simulink model "Final_EWASP_VC"  (R2022a)
settings: Solver=ode1  StartTime=0.0  StopTime=24*3600  FixedStep=10  RelTol=1e-3
values from neighbouring files (symbols this model uses):
  Aux_Threshold = 52    [Setup_Code_EWASP_VC.m]
  buildingAge = 2005    [Setup_Code_EWASP_VC.m]
  ceilingHeight = 2.4    [Setup_Code_EWASP_VC.m]
  conductiveHconnectMatrix = [ ... (first row only)    [Setup_Code_EWASP_VC.m]
  cRoofGreen = 100000    [Setup_Code_EWASP_VC.m]
  Defrost_After_Time = 30    [Setup_Code_EWASP_VC.m]
  DHWDemandProfile = occFreegainHotwaterElecTestPassiveOcc3(:,3)    [Setup_Code_EWASP_VC.m]
  Elec_Max = Elec_Max*(30/24.2)    [Setup_Code_EWASP_VC.m]
  Elec_Mid = Elec_Mid*(30/24.2)    [Setup_Code_EWASP_VC.m]
  Elec_Min = Elec_Min*(30/24.2)    [Setup_Code_EWASP_VC.m]
  ElecDemandProfile = occFreegainHotwaterElecTestPassiveOcc3(:,4)    [Setup_Code_EWASP_VC.m]
  ElecFixed = [Elec_Max(6,2) Elec_Max(6,4) Elec_Max(6,6) Elec_Max(6,7) ... (first row only)    [Setup_Code_EWASP_VC.m]
  floorOrCeilingArea = floorOrCeilingArea*1.15    [Setup_Code_EWASP_VC.m]
  forceCold = 0    [Setup_Code_EWASP_VC.m]
  freegain = occFreegainHotwaterElecTestPassiveOcc3(:,2)-max(occupancy)*25    [Setup_Code_EWASP_VC.m]
  furnitureModelOn = 1    [Setup_Code_EWASP_VC.m]
  Heat_Max = Heat_Max*(30/24.2)    [Setup_Code_EWASP_VC.m]
  Heat_Mid = Heat_Mid*(30/24.2)    [Setup_Code_EWASP_VC.m]
  Heat_Min = Heat_Min*(30/24.2)    [Setup_Code_EWASP_VC.m]
  HeatFixed = [Heat_Max(6,2) Heat_Max(6,4) Heat_Max(6,6) Heat_Max(6,7) ... (first row only)    [Setup_Code_EWASP_VC.m]
  HeatingOnProfile = repmat(HeatingOnProfile,365,1)    [Setup_Code_EWASP_VC.m]
  HEX_ReturnLowerLimit = 52.5    [Setup_Code_EWASP_VC.m]
  HEX_ReturnUpperLimit = 55    [Setup_Code_EWASP_VC.m]
  LeakMultiplier = 1+(2*(rand()-0.5)/10)    [Setup_Code_EWASP_VC.m]
  loopCap = 15    [Setup_Code_EWASP_VC.m]
  maxOcc = max(occupancyProfile)    [Setup_Code_EWASP_VC.m]
  NESW_wallArea = max(NESW_Lengths*ceilingHeight-NESW_Windows,0)    [Setup_Code_EWASP_VC.m]
  NESW_Windows = [ ... (first row only)    [Setup_Code_EWASP_VC.m]
  numRooms = roomCount    [Setup_Code_EWASP_VC.m]
  offsetDays = 0    [Setup_Code_EWASP_VC.m]
  pumpChoice = pumpChoices(MinIndex,1)    [Setup_Code_EWASP_VC.m]
  pumpRamp = 180    [Setup_Code_EWASP_VC.m]
  ReturnLowerLimit = 37.5    [Setup_Code_EWASP_VC.m]
  ReturnUpperLimit = 40    [Setup_Code_EWASP_VC.m]
  RoofIrradiance = Flat_NS_EW_RoofIrradiance(:,1)    [Setup_Code_EWASP_VC.m]
  roofStartTemp = ones(11,1)*20    [Setup_Code_EWASP_VC.m]
  rooftype = 0    [Setup_Code_EWASP_VC.m]
  RoomDataMatrix = [zeros(1,12);ones(1,12)*wallDensity;zeros(1,12);ones(1,12)*wallU;ones(1,12)*windowU;ones(1,12)*floorU;ones(1,12)*ceilingU;zeros(1,12);windowArea, 0;floorOrCeilingArea;zeros(1,12);floorOrCeilingArea*ceilingHeight]    [Setup_Code_EWASP_VC.m]
  roomVol = roomVol*1.15    [Setup_Code_EWASP_VC.m]
  slabStartTemp = (GroundTempTimeSeries(offsetDays*1440+1,1)+thermostatSetting)/2    [Setup_Code_EWASP_VC.m]
  SlackRequest = zeros(1440,1)    [Setup_Code_EWASP_VC.m]
  SolarThermalExists = 0    [Setup_Code_EWASP_VC.m]
  SourceFixed = HeatFixed-ElecFixed    [Setup_Code_EWASP_VC.m]
  StateSeries = StateSeriesGenerator(22,7,1)    [Setup_Code_EWASP_VC.m]
  Tank_Lower_Temp = 49.5    [Setup_Code_EWASP_VC.m]
  Tank_Upper_Temp = 52    [Setup_Code_EWASP_VC.m]
  Tank_Volume_m3 = 0.15    [Setup_Code_EWASP_VC.m]
  TankHeatHour = randi([1 5])-1    [Setup_Code_EWASP_VC.m]
  thermostatSetting = 20.0    (= 20)    [Setup_Code_EWASP_VC.m]
  upDown = [0;0;0;0;1;1;1;1;1;1;1]    [Setup_Code_EWASP_VC.m]
  variableASHP = 1    [Setup_Code_EWASP_VC.m]
  wallStartTempExt = thermostatSetting*(0.266+0.00215*outdoorStartTemp+0.018*wallU+0.00113*outdoorStartTemp*wallU+0.0068*wallU^2)    [Setup_Code_EWASP_VC.m]
undefined symbols (not defined in the file or in its folder): a, ceilingU, condUDMatrix, convUDMatrix, deltaPEXPANDED_E, deltaPEXPANDED_E2, deltaPEXPANDED_N, deltaPEXPANDED_N2, deltaPEXPANDED_S, deltaPEXPANDED_S2, deltaPEXPANDED_W, deltaPEXPANDED_W2, DesiredDHWTemp, DesiredFlowTempVsInOutDeltaTemp, DiffuseHorizontal, DiscIntNeverNeededParam, DNI, dwnAndConcrete, DWORK_A_HX, DWORK_CHK_FLU, DWORK_CP_NODE, DWORK_DH, DWORK_FLUID, DWORK_HCON, DWORK_LOSS, DWORK_MDOTDOWN, DWORK_MDOTIN, DWORK_MDOTUP, DWORK_MIX, DWORK_PRESS, DWORK_QDOTIN, DWORK_RHO_NODE, DWORK_TIN, DWORK_TS_OLD, DWORK_V_NODE, GroundTempTimeSeries, HCM, HCM2, HCM_closed, HCM_closed2, intermediateU, IsTop, massFlowMatrix, neighbourMatrix, numericalRoomUse, RadiatorMatrix, room2roomflowmatrix_E, room2roomflowmatrix_E2, room2roomflowmatrix_N, room2roomflowmatrix_N2, room2roomflowmatrix_S, room2roomflowmatrix_S2, room2roomflowmatrix_W, room2roomflowmatrix_W2, StateAirInEXPANDED_E, StateAirInEXPANDED_E2, StateAirInEXPANDED_N, StateAirInEXPANDED_N2, StateAirInEXPANDED_S, StateAirInEXPANDED_S2 ... (+23)
libraries: simulink x6, dspsigops x4, dspmtrx3 x4, carnot x3, spsEdgeDetectorLib x2, dspstat3 x2, powerlib_meascontrol x1, simulink_extras x1
(part 23 of 27)

== system Final_EWASP_VC/ASHP_Subsystem_Variable/DHW for ASHP Case/HeatPump_Simplified2/HeatPump_basic/model hot side ==
  note: Qdot_h = K1*Tcold_in + K2*Thot_out + K3
      |
      | Qdot_c = -K7*Tcold_in - K8*Thot_out - K9
      |
      | cap_h*dTh/dt = Qdot_h + mdot_h*cp_h*(Th_in-Th) + UA*(Tamb-Th)
      |
      | cap_c*dTc/dt = Qdot_c + mdot_c*cp_c*(Tc_in-Tc) + UA*(Tamb-Tc)
      |
      | cap_h = mass_hot_side * heat_capactiy_hot_side
      |
      | cap_c = mass_cold_side * heat_capactiy_cold_side
  Tcold : Inport
  Thot : Inport  Port=2
  mdot_hot : Inport  Port=3
  Tamb : Inport  Port=4
  command : Inport  Port=5
  Defrost Delta In : Inport  Port=6
  1/(m*cp) : Gain  Gain=1/caph
  Add1 : Sum
  Add2 : Sum  Inputs=+-
  Add4 : Sum  Inputs=+-
  Bias : Bias  Bias=1  SaturateOnIntegerOverflow=off
  Constant : Constant  Value=4180
  Constant1 : Constant  Value=50
  Discrete-Time Integrator : DiscreteIntegrator  InitialConditionSource=external  SampleTime=-1  ICPrevOutput=DiscIntNeverNeededParam  ICPrevScaledInput=DiscIntNeverNeededParam
  Display{,1..5} (6 alike) : Display
  Product{2..5} (4 alike) : DotProduct  OutDataTypeStr=Inherit: Inherit via internal rule
  Scope : Scope
  Scope1 : Scope
  Sum1 : Sum  Inputs=+++  InputSameDT=on  SaturateOnIntegerOverflow=on  OutDataTypeStr=Inherit: Same as first input
  Sum2 : Sum  Inputs=+++  InputSameDT=on  SaturateOnIntegerOverflow=on  OutDataTypeStr=Inherit: Same as first input
  Thot_dependancy : Gain  Gain=K(2)  SaturateOnIntegerOverflow=on  OutDataTypeStr=Inherit: Same as input  ParamDataTypeStr=Inherit: Same as input
  Tsource dependancy : Gain  Gain=K(1)  SaturateOnIntegerOverflow=on  OutDataTypeStr=Inherit: Same as input  ParamDataTypeStr=Inherit: Same as input
  const Power1 : Gain  Gain=-1  SaturateOnIntegerOverflow=on  OutDataTypeStr=Inherit: Same as input  ParamDataTypeStr=Inherit: Same as input
  constant power : Constant  Value=K(3)
  losses : Gain  Gain=UA
  mdot*cp : Outport  VectorParamsAs1DForOutWhenUnconnected=off
  Thot_out : Outport  Port=2  VectorParamsAs1DForOutWhenUnconnected=off
  Real P_therm : Outport  Port=3  VectorParamsAs1DForOutWhenUnconnected=off
  Main Delta : Outport  Port=4  VectorParamsAs1DForOutWhenUnconnected=off
  wires:
  Thot/1 -> Display1/1, Add4/1
  Product2/1 -> mdot*cp/1, Product5/1
  Constant/1 -> Product2/2
  mdot_hot/1 -> Display/1, Product2/1
  Add2/1 -> losses/1
  Tcold/1 -> Display3/1, Tsource dependancy/1
  Tsource dependancy/1 -> Sum1/1
  Thot_dependancy/1 -> Sum1/2
  constant power/1 -> Sum1/3
  Sum1/1 -> Display5/1, Product4/2  "Qdot_hot"
  Tamb/1 -> Display4/1, Add2/1
  command/1 -> Display2/1, Product4/1, const Power1/1
  losses/1 -> Product3/2
  Bias/1 -> Product3/1
  const Power1/1 -> Bias/1
  Add4/1 -> Product5/2
  Sum2/1 -> 1/(m*cp)/1
  Product3/1 -> Sum2/3
  Product4/1 -> Real P_therm/1, Sum2/2
  Product5/1 -> Sum2/1
  Discrete-Time Integrator/1 -> Thot_out/1, Add4/2, Thot_dependancy/1, Add2/2, Scope/1
  1/(m*cp)/1 -> Add1/1, Main Delta/1, Scope1/1
  Add1/1 -> Discrete-Time Integrator/1
  Defrost Delta In/1 -> Add1/2
  Constant1/1 -> Discrete-Time Integrator/2

== system Final_EWASP_VC/ASHP_Subsystem_Variable/DHW for ASHP Case/Storage_Type_2_CONF/HX_EN12977_1/sfun_storage_heatexchanger ==
  Tnodes : Inport
  Temperature : Inport  Port=2
  MassFlow : Inport  Port=3
  Ground : Ground
  Ground1 : Ground
  Ground2 : Ground
  Mux1 : Mux  Inputs=5
  storeHX1 : S-Function  FunctionName=storage_heatexchangerMOD  Parameters=id, nodes, inlet, outlet, p1, p2, p3, p4, p5, p6, p7  SFunctionDeploymentMode=off  EnableBusSupport=off  SFcnStateName=DWORK_TS_OLD,DWORK_A_HX
      settings: SFcnIsStateOwnerBlock=on
  Qnodes : Outport  VectorParamsAs1DForOutWhenUnconnected=off
  Thx : Outport  Port=2  VectorParamsAs1DForOutWhenUnconnected=off
  wires:
  Mux1/1 -> storeHX1/2
  Temperature/1 -> Mux1/1
  Tnodes/1 -> storeHX1/1
  storeHX1/1 -> Qnodes/1
  storeHX1/2 -> Thx/1
  Ground/1 -> Mux1/3
  Ground1/1 -> Mux1/4
  Ground2/1 -> Mux1/5
  MassFlow/1 -> Mux1/2

== system Final_EWASP_VC/Airflow Model/Subsystem1/Subsystem/Subsystem1/average density of air between rooms represented by row and column ==
  In1 : Inport
  In2 : Inport  Port=2
  Constant : Constant  Value=2
  Divide : Product  Inputs=*/
  Minus1 : Sum
  Out1 : Outport  VectorParamsAs1DForOutWhenUnconnected=off
  wires:
  Minus1/1 -> Divide/1
  Constant/1 -> Divide/2
  In2/1 -> Minus1/2
  Divide/1 -> Out1/1
  In1/1 -> Minus1/1

== system Final_EWASP_VC/Airflow Model/Subsystem2/Subsystem/Subsystem1/average density of air between rooms represented by row and column ==
  In1 : Inport
  In2 : Inport  Port=2
  Constant : Constant  Value=2
  Divide : Product  Inputs=*/
  Minus1 : Sum
  Out1 : Outport  VectorParamsAs1DForOutWhenUnconnected=off
  wires:
  Minus1/1 -> Divide/1
  Constant/1 -> Divide/2
  In2/1 -> Minus1/2
  Divide/1 -> Out1/1
  In1/1 -> Minus1/1

== system Final_EWASP_VC/GSHP_Subsystem/DHW for GSHP case/HeatPump_Simplified/HeatPump_basic/P_el calculus ==
  note: Pel = K4*Tcold_in + K5*Thot_out + K6
  Thot_out : Inport
  Tcold_in : Inport  Port=2
  Add : Sum  Inputs=+++
  Thot_dependancy : Gain  Gain=K(5)  SaturateOnIntegerOverflow=on  OutDataTypeStr=Inherit: Same as input  ParamDataTypeStr=Inherit: Same as input
  Tsource dependancy : Gain  Gain=K(4)  SaturateOnIntegerOverflow=on  OutDataTypeStr=Inherit: Same as input  ParamDataTypeStr=Inherit: Same as input
  constant power : Constant  Value=K(6)
  P_el : Outport  VectorParamsAs1DForOutWhenUnconnected=off
  wires:
  constant power/1 -> Add/3
  Tcold_in/1 -> Tsource dependancy/1
  Add/1 -> P_el/1
  Tsource dependancy/1 -> Add/2
  Thot_out/1 -> Thot_dependancy/1
  Thot_dependancy/1 -> Add/1

== system Final_EWASP_VC/GSHP_Subsystem/DHW for GSHP case/HeatPump_Simplified/HeatPump_basic/model cold side ==
  note: Qdot_h = K1*Tcold_in + K2*Thot_out + K3
      |
      | Qdot_c = -K7*Tcold_in - K8*Thot_out - K9
      |
      | cap_h*dTh/dt = Qdot_h + mdot_h*cp_h*(Th_in-Th) + UA*(Tamb-Th)
      |
      | cap_c*dTc/dt = Qdot_c + mdot_c*cp_c*(Tc_in-Tc) + UA*(Tamb-Tc)
      |
      | cap_h = mass_hot_side * heat_capactiy_hot_side
      |
      | cap_c = mass_cold_side * heat_capactiy_cold_side
  Tcold : Inport
  mdot_cold : Inport  Port=2
  Thot : Inport  Port=3
  Tamb : Inport  Port=4
  command : Inport  Port=5
  1/(m*cp) : Gain  Gain=1/capc
  Add2 : Sum  Inputs=+-
  Add4 : Sum  Inputs=+-
  Constant : Constant  Value=4180
  Integrator : Integrator  InitialConditionSource=external  InitialCondition=25
  Product{2..5} (4 alike) : DotProduct  OutDataTypeStr=Inherit: Inherit via internal rule
  Sum1 : Sum  Inputs=---  InputSameDT=on  SaturateOnIntegerOverflow=on  OutDataTypeStr=Inherit: Same as first input
  Sum2 : Sum  Inputs=3  InputSameDT=on  SaturateOnIntegerOverflow=on  OutDataTypeStr=Inherit: Same as first input
  Thot_dependancy : Gain  Gain=K(8)  SaturateOnIntegerOverflow=on  OutDataTypeStr=Inherit: Same as input  ParamDataTypeStr=Inherit: Same as input
  Tsource dependancy : Gain  Gain=K(7)  SaturateOnIntegerOverflow=on  OutDataTypeStr=Inherit: Same as input  ParamDataTypeStr=Inherit: Same as input
  add constant : Subsystem  mask(add constant){c=+1}
      mask prompts: c "constant c"
      mask help: This block adds a constant c to each element of the input vector.
      mask Help: eval('htmlhelp (''chap_4_2a.htm#add_constant'')')
      mask Display: disp('+c');
  const Power1 : Gain  Gain=-1  SaturateOnIntegerOverflow=on  OutDataTypeStr=Inherit: Same as input  ParamDataTypeStr=Inherit: Same as input
  constant power : Constant  Value=K(9)
  losses : Gain  Gain=UA
  Tcold_out : Outport  VectorParamsAs1DForOutWhenUnconnected=off
  mdot*cp : Outport  Port=2  VectorParamsAs1DForOutWhenUnconnected=off
  wires:
  Integrator/1 -> Add4/2, Add2/2, Tcold_out/1
  Product5/1 -> Sum2/1
  Product4/1 -> Sum2/2
  Product3/1 -> Sum2/3
  Sum2/1 -> 1/(m*cp)/1
  Add4/1 -> Product5/2
  const Power1/1 -> add constant/1(In1)
  add constant/1(Out1) -> Product3/1
  losses/1 -> Product3/2
  command/1 -> const Power1/1, Product4/1
  Tamb/1 -> Integrator/2, Add2/1
  Sum1/1 -> Product4/2  "Qdot_hot"
  constant power/1 -> Sum1/3
  Thot_dependancy/1 -> Sum1/2
  Tsource dependancy/1 -> Sum1/1
  Tcold/1 -> Tsource dependancy/1, Add4/1
  Add2/1 -> losses/1
  mdot_cold/1 -> Product2/1
  Product2/1 -> mdot*cp/1, Product5/1
  Thot/1 -> Thot_dependancy/1
  1/(m*cp)/1 -> Integrator/1
  Constant/1 -> Product2/2

== system Final_EWASP_VC/GSHP_Subsystem/DHW for GSHP case/HeatPump_Simplified/HeatPump_basic/model hot side ==
  note: Qdot_h = K1*Tcold_in + K2*Thot_out + K3
      |
      | Qdot_c = -K7*Tcold_in - K8*Thot_out - K9
      |
      | cap_h*dTh/dt = Qdot_h + mdot_h*cp_h*(Th_in-Th) + UA*(Tamb-Th)
      |
      | cap_c*dTc/dt = Qdot_c + mdot_c*cp_c*(Tc_in-Tc) + UA*(Tamb-Tc)
      |
      | cap_h = mass_hot_side * heat_capactiy_hot_side
      |
      | cap_c = mass_cold_side * heat_capactiy_cold_side
  Tcold : Inport
  Thot : Inport  Port=2
  mdot_hot : Inport  Port=3
  Tamb : Inport  Port=4
  command : Inport  Port=5
  1/(m*cp) : Gain  Gain=1/caph
  Add2 : Sum  Inputs=+-
  Add4 : Sum  Inputs=+-
  Bias : Bias  Bias=1  SaturateOnIntegerOverflow=off
  Constant : Constant  Value=4180
  Constant1 : Constant  Value=50
  Discrete-Time Integrator : DiscreteIntegrator  InitialConditionSource=external  SampleTime=-1  ICPrevOutput=DiscIntNeverNeededParam  ICPrevScaledInput=DiscIntNeverNeededParam
  Product{2..5} (4 alike) : DotProduct  OutDataTypeStr=Inherit: Inherit via internal rule
  Sum1 : Sum  Inputs=+++  InputSameDT=on  SaturateOnIntegerOverflow=on  OutDataTypeStr=Inherit: Same as first input
  Sum2 : Sum  Inputs=+++  InputSameDT=on  SaturateOnIntegerOverflow=on  OutDataTypeStr=Inherit: Same as first input
  Thot_dependancy : Gain  Gain=K(2)  SaturateOnIntegerOverflow=on  OutDataTypeStr=Inherit: Same as input  ParamDataTypeStr=Inherit: Same as input
  Tsource dependancy : Gain  Gain=K(1)  SaturateOnIntegerOverflow=on  OutDataTypeStr=Inherit: Same as input  ParamDataTypeStr=Inherit: Same as input
  const Power1 : Gain  Gain=-1  SaturateOnIntegerOverflow=on  OutDataTypeStr=Inherit: Same as input  ParamDataTypeStr=Inherit: Same as input
  constant power : Constant  Value=K(3)
  losses : Gain  Gain=UA
  mdot*cp : Outport  VectorParamsAs1DForOutWhenUnconnected=off
  Thot_out : Outport  Port=2  VectorParamsAs1DForOutWhenUnconnected=off
  Real P_therm : Outport  Port=3  VectorParamsAs1DForOutWhenUnconnected=off
  wires:
  Thot/1 -> Add4/1
  Product2/1 -> mdot*cp/1, Product5/1
  Constant/1 -> Product2/2
  mdot_hot/1 -> Product2/1
  Add2/1 -> losses/1
  Tcold/1 -> Tsource dependancy/1
  Tsource dependancy/1 -> Sum1/1
  Thot_dependancy/1 -> Sum1/2
  constant power/1 -> Sum1/3
  Sum1/1 -> Product4/2  "Qdot_hot"
  Tamb/1 -> Add2/1
  command/1 -> Product4/1, const Power1/1
  losses/1 -> Product3/2
  Bias/1 -> Product3/1
  const Power1/1 -> Bias/1
  Add4/1 -> Product5/2
  Sum2/1 -> 1/(m*cp)/1
  1/(m*cp)/1 -> Discrete-Time Integrator/1
  Product3/1 -> Sum2/3
  Product4/1 -> Real P_therm/1, Sum2/2
  Product5/1 -> Sum2/1
  Discrete-Time Integrator/1 -> Thot_out/1, Add4/2, Thot_dependancy/1, Add2/2
  Constant1/1 -> Discrete-Time Integrator/2

== system Final_EWASP_VC/GSHP_Subsystem/DHW for GSHP case/Storage_Type_2_CONF/HX_EN12977_1/sfun_storage_heatexchanger ==
  Tnodes : Inport
  Temperature : Inport  Port=2
  MassFlow : Inport  Port=3
  Ground : Ground
  Ground1 : Ground
  Ground2 : Ground
  Mux1 : Mux  Inputs=5
  storeHX1 : S-Function  FunctionName=storage_heatexchangerMOD  Parameters=id, nodes, inlet, outlet, p1, p2, p3, p4, p5, p6, p7  SFunctionDeploymentMode=off  EnableBusSupport=off  SFcnStateName=DWORK_TS_OLD
      settings: SFcnIsStateOwnerBlock=on
  Qnodes : Outport  VectorParamsAs1DForOutWhenUnconnected=off
  Thx : Outport  Port=2  VectorParamsAs1DForOutWhenUnconnected=off
  wires:
  Mux1/1 -> storeHX1/2
  Temperature/1 -> Mux1/1
  Tnodes/1 -> storeHX1/1
  storeHX1/1 -> Qnodes/1
  storeHX1/2 -> Thx/1
  Ground/1 -> Mux1/3
  Ground1/1 -> Mux1/4
  Ground2/1 -> Mux1/5
  MassFlow/1 -> Mux1/2

== system Final_EWASP_VC/GSHP_Subsystem/Subsystem3/Ground_Source_Heat_Exchanger1/Randbedingung 2/g-function ==
  note: Trichter: 1/(4*pi*lambdaErde)
  T(i,1)-T(i,0) : Inport
  Constant : Constant  Value=t_start
  Dd1 : Gain  Gain=L1/(Ts_Trichter*Dl)  SaturateOnIntegerOverflow=on  OutDataTypeStr=Inherit: Same as input  ParamDataTypeStr=Inherit: Same as input
  Dd2 : Gain  Gain=1/(2*pi*lambdaErde)  SaturateOnIntegerOverflow=on  OutDataTypeStr=Inherit: Same as input  ParamDataTypeStr=Inherit: Same as input
  Digital Clock : DigitalClock  SampleTime=10
  Integrator : Integrator  ExternalReset=rising
  Product : Product  InputSameDT=on  RndMeth=Zero  SaturateOnIntegerOverflow=on  OutDataTypeStr=Inherit: Same as first input
  Pulse Generator : DiscretePulseGenerator  PulseType=Time based  Period=Ts_Trichter  PulseWidth=50  PhaseDelay=300
  RechenRadius : Constant  Value=Rechenradius  VectorParams1D=off
  Sum : Sum  Inputs=|+-  InputSameDT=on  SaturateOnIntegerOverflow=on  OutDataTypeStr=Inherit: Same as first input
  Sum1 : Sum  Inputs=++|  InputSameDT=on  SaturateOnIntegerOverflow=on  OutDataTypeStr=Inherit: Same as first input
  Sum4 : Sum  Inputs=|++  InputSameDT=on  SaturateOnIntegerOverflow=on  OutDataTypeStr=Inherit: Same as first input
  Unit Delay : UnitDelay  SampleTime=10  HasFrameUpgradeWarning=on
  Unit Delay1 : UnitDelay  SampleTime=10  HasFrameUpgradeWarning=on
  Zero-Order Hold2 : ZeroOrderHold  SampleTime=10
  Zero-Order Hold3 : ZeroOrderHold  SampleTime=10
  g-function : Lookup2D  RowIndex=t_Trichter  ColumnIndex=r_Trichter  Table=gfunction
  DeltaT : Outport  VectorParamsAs1DForOutWhenUnconnected=off
  wires:
  Constant/1 -> Sum1/1
  Sum1/1 -> g-function/1
  Digital Clock/1 -> Sum1/2
  Pulse Generator/1 -> Integrator/2
  Integrator/1 -> Dd1/1
  Dd1/1 -> Zero-Order Hold2/1
  Unit Delay/1 -> Sum/2
  Sum/1 -> Product/1
  g-function/1 -> Dd2/1
  RechenRadius/1 -> Zero-Order Hold3/1
  Product/1 -> Sum4/1
  Dd2/1 -> Product/2
  Unit Delay1/1 -> Sum4/2
  Sum4/1 -> Unit Delay1/1, DeltaT/1
  Zero-Order Hold3/1 -> g-function/2
  Zero-Order Hold2/1 -> Unit Delay/1, Sum/1
  T(i,1)-T(i,0)/1 -> Integrator/1

== system Final_EWASP_VC/GSHP_Subsystem/Subsystem3/HeatPump_Simplified/HeatPump_basic/P_el calculus ==
  note: Pel = K4*Tcold_in + K5*Thot_out + K6
  Thot_out : Inport
  Tcold_in : Inport  Port=2
  Add : Sum  Inputs=+++
  Thot_dependancy : Gain  Gain=K(5)  SaturateOnIntegerOverflow=on  OutDataTypeStr=Inherit: Same as input  ParamDataTypeStr=Inherit: Same as input
  Tsource dependancy : Gain  Gain=K(4)  SaturateOnIntegerOverflow=on  OutDataTypeStr=Inherit: Same as input  ParamDataTypeStr=Inherit: Same as input
  constant power : Constant  Value=K(6)
  P_el : Outport  VectorParamsAs1DForOutWhenUnconnected=off
  wires:
  constant power/1 -> Add/3
  Tcold_in/1 -> Tsource dependancy/1
  Add/1 -> P_el/1
  Tsource dependancy/1 -> Add/2
  Thot_out/1 -> Thot_dependancy/1
  Thot_dependancy/1 -> Add/1

== system Final_EWASP_VC/GSHP_Subsystem/Subsystem3/HeatPump_Simplified/HeatPump_basic/model cold side ==
  note: Qdot_h = K1*Tcold_in + K2*Thot_out + K3
      |
      | Qdot_c = -K7*Tcold_in - K8*Thot_out - K9
      |
      | cap_h*dTh/dt = Qdot_h + mdot_h*cp_h*(Th_in-Th) + UA*(Tamb-Th)
      |
      | cap_c*dTc/dt = Qdot_c + mdot_c*cp_c*(Tc_in-Tc) + UA*(Tamb-Tc)
      |
      | cap_h = mass_hot_side * heat_capactiy_hot_side
      |
      | cap_c = mass_cold_side * heat_capactiy_cold_side
  Tcold : Inport
  mdot_cold : Inport  Port=2
  Thot : Inport  Port=3
  Tamb : Inport  Port=4
  command : Inport  Port=5
  1/(m*cp) : Gain  Gain=1/capc
  Add2 : Sum  Inputs=+-
  Add4 : Sum  Inputs=+-
  Constant : Constant  Value=4180
  Integrator : Integrator  InitialConditionSource=external  InitialCondition=25
  Product{2..5} (4 alike) : DotProduct  OutDataTypeStr=Inherit: Inherit via internal rule
  Sum1 : Sum  Inputs=---  InputSameDT=on  SaturateOnIntegerOverflow=on  OutDataTypeStr=Inherit: Same as first input
  Sum2 : Sum  Inputs=3  InputSameDT=on  SaturateOnIntegerOverflow=on  OutDataTypeStr=Inherit: Same as first input
  Thot_dependancy : Gain  Gain=K(8)  SaturateOnIntegerOverflow=on  OutDataTypeStr=Inherit: Same as input  ParamDataTypeStr=Inherit: Same as input
  Tsource dependancy : Gain  Gain=K(7)  SaturateOnIntegerOverflow=on  OutDataTypeStr=Inherit: Same as input  ParamDataTypeStr=Inherit: Same as input
  add constant : Subsystem  mask(add constant){c=+1}
      mask prompts: c "constant c"
      mask help: This block adds a constant c to each element of the input vector.
      mask Help: eval('htmlhelp (''chap_4_2a.htm#add_constant'')')
      mask Display: disp('+c');
  const Power1 : Gain  Gain=-1  SaturateOnIntegerOverflow=on  OutDataTypeStr=Inherit: Same as input  ParamDataTypeStr=Inherit: Same as input
  constant power : Constant  Value=K(9)
  losses : Gain  Gain=UA
  Tcold_out : Outport  VectorParamsAs1DForOutWhenUnconnected=off
  mdot*cp : Outport  Port=2  VectorParamsAs1DForOutWhenUnconnected=off
  wires:
  Integrator/1 -> Add4/2, Add2/2, Tcold_out/1
  Product5/1 -> Sum2/1
  Product4/1 -> Sum2/2
  Product3/1 -> Sum2/3
  Sum2/1 -> 1/(m*cp)/1
  Add4/1 -> Product5/2
  const Power1/1 -> add constant/1(In1)
  add constant/1(Out1) -> Product3/1
  losses/1 -> Product3/2
  command/1 -> const Power1/1, Product4/1
  Tamb/1 -> Integrator/2, Add2/1
  Sum1/1 -> Product4/2  "Qdot_hot"
  constant power/1 -> Sum1/3
  Thot_dependancy/1 -> Sum1/2
  Tsource dependancy/1 -> Sum1/1
  Tcold/1 -> Tsource dependancy/1, Add4/1
  Add2/1 -> losses/1
  mdot_cold/1 -> Product2/1
  Product2/1 -> mdot*cp/1, Product5/1
  Thot/1 -> Thot_dependancy/1
  1/(m*cp)/1 -> Integrator/1
  Constant/1 -> Product2/2

== system Final_EWASP_VC/GSHP_Subsystem/Subsystem3/HeatPump_Simplified/HeatPump_basic/model hot side ==
  note: Qdot_h = K1*Tcold_in + K2*Thot_out + K3
      |
      | Qdot_c = -K7*Tcold_in - K8*Thot_out - K9
      |
      | cap_h*dTh/dt = Qdot_h + mdot_h*cp_h*(Th_in-Th) + UA*(Tamb-Th)
      |
      | cap_c*dTc/dt = Qdot_c + mdot_c*cp_c*(Tc_in-Tc) + UA*(Tamb-Tc)
      |
      | cap_h = mass_hot_side * heat_capactiy_hot_side
      |
      | cap_c = mass_cold_side * heat_capactiy_cold_side
  Tcold : Inport
  Thot : Inport  Port=2
  mdot_hot : Inport  Port=3
  Tamb : Inport  Port=4
  command : Inport  Port=5
  Tamb1 : Inport  Port=6
  1/(m*cp) : Gain  Gain=1/caph
  Add2 : Sum  Inputs=+-
  Add4 : Sum  Inputs=+-
  Bias : Bias  Bias=1  SaturateOnIntegerOverflow=off
  Constant : Constant  Value=4180
  Integrator : Integrator  InitialConditionSource=external  InitialCondition=25
  Product : Product
  Product{2..5} (4 alike) : DotProduct  OutDataTypeStr=Inherit: Inherit via internal rule
  Sum1 : Sum  Inputs=+++  InputSameDT=on  SaturateOnIntegerOverflow=on  OutDataTypeStr=Inherit: Same as first input
  Sum2 : Sum  Inputs=+++  InputSameDT=on  SaturateOnIntegerOverflow=on  OutDataTypeStr=Inherit: Same as first input
  Thot_dependancy : Gain  Gain=K(2)  SaturateOnIntegerOverflow=on  OutDataTypeStr=Inherit: Same as input  ParamDataTypeStr=Inherit: Same as input
  Tsource dependancy : Gain  Gain=K(1)  SaturateOnIntegerOverflow=on  OutDataTypeStr=Inherit: Same as input  ParamDataTypeStr=Inherit: Same as input
  const Power1 : Gain  Gain=-1  SaturateOnIntegerOverflow=on  OutDataTypeStr=Inherit: Same as input  ParamDataTypeStr=Inherit: Same as input
  constant power : Constant  Value=K(3)
  losses : Gain  Gain=UA
  mdot*cp : Outport  VectorParamsAs1DForOutWhenUnconnected=off
  Thot_out : Outport  Port=2  VectorParamsAs1DForOutWhenUnconnected=off
  Real P_therm : Outport  Port=3  VectorParamsAs1DForOutWhenUnconnected=off
  wires:
  Thot/1 -> Add4/1
  Product2/1 -> mdot*cp/1, Product5/1
  Constant/1 -> Product2/2
  mdot_hot/1 -> Product2/1
  Add2/1 -> losses/1
  Tcold/1 -> Tsource dependancy/1
  Tsource dependancy/1 -> Sum1/1
  Thot_dependancy/1 -> Sum1/2
  constant power/1 -> Sum1/3
  Sum1/1 -> Product/1  "Qdot_hot"
  Tamb/1 -> Add2/1, Integrator/2
  command/1 -> Product4/1, const Power1/1
  losses/1 -> Product3/2
  Bias/1 -> Product3/1
  const Power1/1 -> Bias/1
  Add4/1 -> Product5/2
  Sum2/1 -> 1/(m*cp)/1
  1/(m*cp)/1 -> Integrator/1
  Product3/1 -> Sum2/3
  Product4/1 -> Real P_therm/1, Sum2/2
  Product5/1 -> Sum2/1
  Integrator/1 -> Thot_out/1, Add4/2, Thot_dependancy/1, Add2/2
  Product/1 -> Product4/2
  Tamb1/1 -> Product/2

== system Final_EWASP_VC/ASHP_Subsystem/DHW for ASHP Case/HeatPump_Simplified1/HeatPump_basic/model cold side/add constant ==
  In1 : Inport
  Sum : Sum  InputSameDT=on  SaturateOnIntegerOverflow=on  OutDataTypeStr=Inherit: Same as first input
  const : Constant  Value=c
  Out1 : Outport  VectorParamsAs1DForOutWhenUnconnected=off
  wires:
  Sum/1 -> Out1/1
  In1/1 -> Sum/2
  const/1 -> Sum/1

== system Final_EWASP_VC/ASHP_Subsystem/DHW for ASHP Case/HeatPump_Simplified2/HeatPump_basic/model cold side/add constant ==
  In1 : Inport
  Sum : Sum  InputSameDT=on  SaturateOnIntegerOverflow=on  OutDataTypeStr=Inherit: Same as first input
  const : Constant  Value=c
  Out1 : Outport  VectorParamsAs1DForOutWhenUnconnected=off
  wires:
  Sum/1 -> Out1/1
  In1/1 -> Sum/2
  const/1 -> Sum/1

== system Final_EWASP_VC/ASHP_Subsystem/Subsystem14/HeatPump_Simplified/HeatPump_basic/model cold side/add constant ==
  In1 : Inport
  Sum : Sum  InputSameDT=on  SaturateOnIntegerOverflow=on  OutDataTypeStr=Inherit: Same as first input
  const : Constant  Value=c
  Out1 : Outport  VectorParamsAs1DForOutWhenUnconnected=off
  wires:
  Sum/1 -> Out1/1
  In1/1 -> Sum/2
  const/1 -> Sum/1

== system Final_EWASP_VC/ASHP_Subsystem/Subsystem14/HeatPump_Simplified1/HeatPump_basic/model cold side/add constant ==
  In1 : Inport
  Sum : Sum  InputSameDT=on  SaturateOnIntegerOverflow=on  OutDataTypeStr=Inherit: Same as first input
  const : Constant  Value=c
  Out1 : Outport  VectorParamsAs1DForOutWhenUnconnected=off
  wires:
  Sum/1 -> Out1/1
  In1/1 -> Sum/2
  const/1 -> Sum/1

== system Final_EWASP_VC/ASHP_Subsystem_Variable/DHW for ASHP Case/HeatPump_Simplified1/HeatPump_basic/model cold side/add constant ==
  In1 : Inport
  Sum : Sum  InputSameDT=on  SaturateOnIntegerOverflow=on  OutDataTypeStr=Inherit: Same as first input
  const : Constant  Value=c
  Out1 : Outport  VectorParamsAs1DForOutWhenUnconnected=off
  wires:
  Sum/1 -> Out1/1
  In1/1 -> Sum/2
  const/1 -> Sum/1

== system Final_EWASP_VC/ASHP_Subsystem_Variable/DHW for ASHP Case/HeatPump_Simplified2/HeatPump_basic/model cold side/add constant ==
  In1 : Inport
  Sum : Sum  InputSameDT=on  SaturateOnIntegerOverflow=on  OutDataTypeStr=Inherit: Same as first input
  const : Constant  Value=c
  Out1 : Outport  VectorParamsAs1DForOutWhenUnconnected=off
  wires:
  Sum/1 -> Out1/1
  In1/1 -> Sum/2
  const/1 -> Sum/1

== system Final_EWASP_VC/GSHP_Subsystem/DHW for GSHP case/HeatPump_Simplified/HeatPump_basic/model cold side/add constant ==
  In1 : Inport
  Sum : Sum  InputSameDT=on  SaturateOnIntegerOverflow=on  OutDataTypeStr=Inherit: Same as first input
  const : Constant  Value=c
  Out1 : Outport  VectorParamsAs1DForOutWhenUnconnected=off
  wires:
  Sum/1 -> Out1/1
  In1/1 -> Sum/2
  const/1 -> Sum/1

== system Final_EWASP_VC/GSHP_Subsystem/Subsystem3/HeatPump_Simplified/HeatPump_basic/model cold side/add constant ==
  In1 : Inport
  Sum : Sum  InputSameDT=on  SaturateOnIntegerOverflow=on  OutDataTypeStr=Inherit: Same as first input
  const : Constant  Value=c
  Out1 : Outport  VectorParamsAs1DForOutWhenUnconnected=off
  wires:
  Sum/1 -> Out1/1
  In1/1 -> Sum/2
  const/1 -> Sum/1

== matlab function Final_EWASP_VC/Subsystem_Room2/Kitchen/Subsystem3/MATLAB Function1 ==
  data: Time input; offsetDays input; SurfaceAlbedo input; Tot_Irradiance output; RoofArea input; c_OutRoof input; deltaTexternal output; RoofIrradiance input
function [Tot_Irradiance, deltaTexternal] = SolarSeriesToExtWallGains(Time,offsetDays,SurfaceAlbedo,RoofArea,c_OutRoof,RoofIrradiance)

PU_AreaIrr=RoofIrradiance(ceil((offsetDays*1440)+Time/60+0.00001),1)/2;%extracts correct Diff for the timestep, factor of 1/2 corrects for 90 degree walls (so only half Diff irradiance can be utilised)


Tot_Irradiance=(RoofArea*PU_AreaIrr)*(1-SurfaceAlbedo);
deltaTexternal=Tot_Irradiance./(c_OutRoof*RoofArea);

    
end

== matlab function Final_EWASP_VC/Subsystem_Room3/Utility/Subsystem3/MATLAB Function ==
  data: uValWall input; deltaTint output; c_InPU input; c_MidPU input; c_OutPU input; T_InWall input; T_MidWall input; T_OutWall input; T_Room input; T_AmbientSeries input; windSpeedSeries input; deltaTmid output; deltaTout output; ceilArea input; roomNumber input; logRoomHeatLoss output; Time input; offsetDays input
function [deltaTint,deltaTmid,deltaTout,logRoomHeatLoss] = fcn(uValWall,c_InPU,c_MidPU,c_OutPU,T_InWall, T_MidWall,T_OutWall,T_Room,T_AmbientSeries,windSpeedSeries,ceilArea,roomNumber,Time,offsetDays)




  deltaTint=zeros(1,1);
   deltaTmid=zeros(1,1);
    deltaTout=zeros(1,1);
    logRoomHeatLoss=zeros(1,1);

    v_Wind=windSpeedSeries(ceil((offsetDays*1440)+Time/60+0.00001),1);
   T_Ambient=T_AmbientSeries(ceil((offsetDays*1440)+Time/60+0.00001),1);
    
k_InMid=uValWall*2;
k_OutMid=uValWall*2;




    
    if ceilArea>0

c_In=c_InPU*ceilArea;
c_Mid=c_MidPU*ceilArea;
c_Out=c_OutPU*ceilArea;

    
aA=[-(k_InMid*ceilArea)/c_In (k_InMid*ceilArea)/c_In 0
 (k_InMid*ceilArea)/c_Mid -((k_InMid+k_OutMid)*ceilArea)/c_Mid (k_OutMid*ceilArea)/c_Mid
 0 (k_OutMid*ceilArea)/c_Out -(k_OutMid*ceilArea)/c_Out];

bA=[1/c_In 0 0
 0 1/c_Mid 0
 0 0 1/c_Out];
    
ab=[T_InWall
    T_MidWall
    T_OutWall];

bb=[(2.5*(T_Room-T_InWall)+5.6*(T_Room-T_InWall))*ceilArea
0    
(2.8+3*v_Wind)*(T_Ambient-T_OutWall)+5.6*(T_Ambient-T_OutWall)*ceilArea];

deltaT=aA*ab+bA*bb;

    deltaTint=deltaT(1,1);
   deltaTmid=deltaT(2,1);
    deltaTout=deltaT(3,1);
    
    logRoomHeatLoss=bb(1,1);
    
    else
        
        deltaTint=0;
   deltaTmid=0;
    deltaTout=0;
        
    logRoomHeatLoss=0;
    
    end

== matlab function Final_EWASP_VC/Subsystem_Room3/Utility/Subsystem3/MATLAB Function1 ==
  data: Time input; offsetDays input; SurfaceAlbedo input; Tot_Irradiance output; RoofArea input; c_OutRoof input; deltaTexternal output; RoofIrradiance input
function [Tot_Irradiance, deltaTexternal] = SolarSeriesToExtWallGains(Time,offsetDays,SurfaceAlbedo,RoofArea,c_OutRoof,RoofIrradiance)

PU_AreaIrr=RoofIrradiance(ceil((offsetDays*1440)+Time/60+0.00001),1)/2;%extracts correct Diff for the timestep, factor of 1/2 corrects for 90 degree walls (so only half Diff irradiance can be utilised)


Tot_Irradiance=(RoofArea*PU_AreaIrr)*(1-SurfaceAlbedo);
deltaTexternal=Tot_Irradiance./(c_OutRoof*RoofArea);

    
end

== matlab function Final_EWASP_VC/Subsystem_Room4/Hall/Subsystem3/MATLAB Function ==
  data: uValWall input; deltaTint output; c_InPU input; c_MidPU input; c_OutPU input; T_InWall input; T_MidWall input; T_OutWall input; T_Room input; T_AmbientSeries input; windSpeedSeries input; deltaTmid output; deltaTout output; ceilArea input; roomNumber input; logRoomHeatLoss output; Time input; offsetDays input
function [deltaTint,deltaTmid,deltaTout,logRoomHeatLoss] = fcn(uValWall,c_InPU,c_MidPU,c_OutPU,T_InWall, T_MidWall,T_OutWall,T_Room,T_AmbientSeries,windSpeedSeries,ceilArea,roomNumber,Time,offsetDays)




  deltaTint=zeros(1,1);
   deltaTmid=zeros(1,1);
    deltaTout=zeros(1,1);
    logRoomHeatLoss=zeros(1,1);

    v_Wind=windSpeedSeries(ceil((offsetDays*1440)+Time/60+0.00001),1);
   T_Ambient=T_AmbientSeries(ceil((offsetDays*1440)+Time/60+0.00001),1);
    
k_InMid=uValWall*2;
k_OutMid=uValWall*2;




    
    if ceilArea>0

c_In=c_InPU*ceilArea;
c_Mid=c_MidPU*ceilArea;
c_Out=c_OutPU*ceilArea;

    
aA=[-(k_InMid*ceilArea)/c_In (k_InMid*ceilArea)/c_In 0
 (k_InMid*ceilArea)/c_Mid -((k_InMid+k_OutMid)*ceilArea)/c_Mid (k_OutMid*ceilArea)/c_Mid
 0 (k_OutMid*ceilArea)/c_Out -(k_OutMid*ceilArea)/c_Out];

bA=[1/c_In 0 0
 0 1/c_Mid 0
 0 0 1/c_Out];
    
ab=[T_InWall
    T_MidWall
    T_OutWall];

bb=[(2.5*(T_Room-T_InWall)+5.6*(T_Room-T_InWall))*ceilArea
0    
(2.8+3*v_Wind)*(T_Ambient-T_OutWall)+5.6*(T_Ambient-T_OutWall)*ceilArea];

deltaT=aA*ab+bA*bb;

    deltaTint=deltaT(1,1);
   deltaTmid=deltaT(2,1);
    deltaTout=deltaT(3,1);
    
    logRoomHeatLoss=bb(1,1);
    
    else
        
        deltaTint=0;
   deltaTmid=0;
    deltaTout=0;
        
    logRoomHeatLoss=0;
    
    end

== matlab function Final_EWASP_VC/Subsystem_Room4/Hall/Subsystem3/MATLAB Function1 ==
  data: Time input; offsetDays input; SurfaceAlbedo input; Tot_Irradiance output; RoofArea input; c_OutRoof input; deltaTexternal output; RoofIrradiance input
function [Tot_Irradiance, deltaTexternal] = SolarSeriesToExtWallGains(Time,offsetDays,SurfaceAlbedo,RoofArea,c_OutRoof,RoofIrradiance)

PU_AreaIrr=RoofIrradiance(ceil((offsetDays*1440)+Time/60+0.00001),1)/2;%extracts correct Diff for the timestep, factor of 1/2 corrects for 90 degree walls (so only half Diff irradiance can be utilised)


Tot_Irradiance=(RoofArea*PU_AreaIrr)*(1-SurfaceAlbedo);
deltaTexternal=Tot_Irradiance./(c_OutRoof*RoofArea);

    
end

== matlab function Final_EWASP_VC/Subsystem_Room5/Landing/Subsystem3/MATLAB Function ==
  data: uValWall input; deltaTint output; c_InPU input; c_MidPU input; c_OutPU input; T_InWall input; T_MidWall input; T_OutWall input; T_Room input; T_AmbientSeries input; windSpeedSeries input; deltaTmid output; deltaTout output; ceilArea input; roomNumber input; logRoomHeatLoss output; Time input; offsetDays input
function [deltaTint,deltaTmid,deltaTout,logRoomHeatLoss] = fcn(uValWall,c_InPU,c_MidPU,c_OutPU,T_InWall, T_MidWall,T_OutWall,T_Room,T_AmbientSeries,windSpeedSeries,ceilArea,roomNumber,Time,offsetDays)




  deltaTint=zeros(1,1);
   deltaTmid=zeros(1,1);
    deltaTout=zeros(1,1);
    logRoomHeatLoss=zeros(1,1);

    v_Wind=windSpeedSeries(ceil((offsetDays*1440)+Time/60+0.00001),1);
   T_Ambient=T_AmbientSeries(ceil((offsetDays*1440)+Time/60+0.00001),1);
    
k_InMid=uValWall*2;
k_OutMid=uValWall*2;




    
    if ceilArea>0

c_In=c_InPU*ceilArea;
c_Mid=c_MidPU*ceilArea;
c_Out=c_OutPU*ceilArea;

    
aA=[-(k_InMid*ceilArea)/c_In (k_InMid*ceilArea)/c_In 0
 (k_InMid*ceilArea)/c_Mid -((k_InMid+k_OutMid)*ceilArea)/c_Mid (k_OutMid*ceilArea)/c_Mid
 0 (k_OutMid*ceilArea)/c_Out -(k_OutMid*ceilArea)/c_Out];

bA=[1/c_In 0 0
 0 1/c_Mid 0
 0 0 1/c_Out];
    
ab=[T_InWall
    T_MidWall
    T_OutWall];

bb=[(2.5*(T_Room-T_InWall)+5.6*(T_Room-T_InWall))*ceilArea
0    
(2.8+3*v_Wind)*(T_Ambient-T_OutWall)+5.6*(T_Ambient-T_OutWall)*ceilArea];

deltaT=aA*ab+bA*bb;

    deltaTint=deltaT(1,1);
   deltaTmid=deltaT(2,1);
    deltaTout=deltaT(3,1);
    
    logRoomHeatLoss=bb(1,1);
    
    else
        
        deltaTint=0;
   deltaTmid=0;
    deltaTout=0;
        
    logRoomHeatLoss=0;
    
    end

== matlab function Final_EWASP_VC/Subsystem_Room5/Landing/Subsystem3/MATLAB Function1 ==
  data: Time input; offsetDays input; SurfaceAlbedo input; Tot_Irradiance output; RoofArea input; c_OutRoof input; deltaTexternal output; RoofIrradiance input
function [Tot_Irradiance, deltaTexternal] = SolarSeriesToExtWallGains(Time,offsetDays,SurfaceAlbedo,RoofArea,c_OutRoof,RoofIrradiance)

PU_AreaIrr=RoofIrradiance(ceil((offsetDays*1440)+Time/60+0.00001),1)/2;%extracts correct Diff for the timestep, factor of 1/2 corrects for 90 degree walls (so only half Diff irradiance can be utilised)


Tot_Irradiance=(RoofArea*PU_AreaIrr)*(1-SurfaceAlbedo);
deltaTexternal=Tot_Irradiance./(c_OutRoof*RoofArea);

    
end

== matlab function Final_EWASP_VC/Subsystem_Room7/Bedroom 2/Subsystem1/MATLAB Function ==
  data: uValWall input; deltaTint output; c_InPU input; c_MidPU input; c_OutPU input; T_InWall input; T_MidWall input; T_OutWall input; T_Room input; T_AmbientSeries input; windSpeedSeries input; deltaTmid output; deltaTout output; ceilArea input; roomNumber input; logRoomHeatLoss output; Time input; offsetDays input
function [deltaTint,deltaTmid,deltaTout,logRoomHeatLoss] = fcn(uValWall,c_InPU,c_MidPU,c_OutPU,T_InWall, T_MidWall,T_OutWall,T_Room,T_AmbientSeries,windSpeedSeries,ceilArea,roomNumber,Time,offsetDays)




  deltaTint=zeros(1,1);
   deltaTmid=zeros(1,1);
    deltaTout=zeros(1,1);
    logRoomHeatLoss=zeros(1,1);

    v_Wind=windSpeedSeries(ceil((offsetDays*1440)+Time/60+0.00001),1);
   T_Ambient=T_AmbientSeries(ceil((offsetDays*1440)+Time/60+0.00001),1);
    
k_InMid=uValWall*2;
k_OutMid=uValWall*2;




    
    if ceilArea>0

c_In=c_InPU*ceilArea;
c_Mid=c_MidPU*ceilArea;
c_Out=c_OutPU*ceilArea;

    
aA=[-(k_InMid*ceilArea)/c_In (k_InMid*ceilArea)/c_In 0
 (k_InMid*ceilArea)/c_Mid -((k_InMid+k_OutMid)*ceilArea)/c_Mid (k_OutMid*ceilArea)/c_Mid
 0 (k_OutMid*ceilArea)/c_Out -(k_OutMid*ceilArea)/c_Out];

bA=[1/c_In 0 0
 0 1/c_Mid 0
 0 0 1/c_Out];
    
ab=[T_InWall
    T_MidWall
    T_OutWall];

bb=[(2.5*(T_Room-T_InWall)+5.6*(T_Room-T_InWall))*ceilArea
0    
(2.8+3*v_Wind)*(T_Ambient-T_OutWall)+5.6*(T_Ambient-T_OutWall)*ceilArea];

deltaT=aA*ab+bA*bb;

    deltaTint=deltaT(1,1);
   deltaTmid=deltaT(2,1);
    deltaTout=deltaT(3,1);
    
    logRoomHeatLoss=bb(1,1);
    
    else
        
        deltaTint=0;
   deltaTmid=0;
    deltaTout=0;
        
    logRoomHeatLoss=0;
    
    end

== matlab function Final_EWASP_VC/Subsystem_Room7/Bedroom 2/Subsystem1/MATLAB Function1 ==
  data: Time input; offsetDays input; SurfaceAlbedo input; Tot_Irradiance output; RoofArea input; c_OutRoof input; deltaTexternal output; RoofIrradiance input
function [Tot_Irradiance, deltaTexternal] = SolarSeriesToExtWallGains(Time,offsetDays,SurfaceAlbedo,RoofArea,c_OutRoof,RoofIrradiance)

PU_AreaIrr=RoofIrradiance(ceil((offsetDays*1440)+Time/60+0.00001),1)/2;%extracts correct Diff for the timestep, factor of 1/2 corrects for 90 degree walls (so only half Diff irradiance can be utilised)


Tot_Irradiance=(RoofArea*PU_AreaIrr)*(1-SurfaceAlbedo);
deltaTexternal=Tot_Irradiance./(c_OutRoof*RoofArea);

    
end

== matlab function Final_EWASP_VC/Subsystem_Room3/Utility/Subsystem1/MATLAB Function ==
  data: uValWall input; deltaTint output; c_InPU input; c_MidPU input; c_OutPU input; T_InWallNEWS input; T_MidWallNEWS input; T_OutWallNEWS input; T_Room input; T_AmbientSeries input; windSpeedSeries input; deltaTmid output; deltaTout output; NESW_wallArea input; roomNumber input; logRoomHeatLoss output; Time input; offsetDays input
function [deltaTint,deltaTmid,deltaTout,logRoomHeatLoss] = fcn(uValWall,c_InPU,c_MidPU,c_OutPU,T_InWallNEWS, T_MidWallNEWS,T_OutWallNEWS,T_Room,T_AmbientSeries,windSpeedSeries,NESW_wallArea,roomNumber,Time,offsetDays)




  deltaTint=zeros(1,4);
   deltaTmid=zeros(1,4);
    deltaTout=zeros(1,4);
    logRoomHeatLoss=zeros(1,4);

    v_Wind=windSpeedSeries(ceil((offsetDays*1440)+Time/60+0.00001),1);
   T_Ambient=T_AmbientSeries(ceil((offsetDays*1440)+Time/60+0.00001),1);
    
k_InMid=uValWall*2;
k_OutMid=uValWall*2;


NEWS_wallArea=NESW_wallArea;
NEWS_wallArea([3 4],:)=NEWS_wallArea([4 3],:);
RoomWallAreas_NEWS=NEWS_wallArea(:,roomNumber)';


for i=1:4
    
    if RoomWallAreas_NEWS(1,i)>0

c_In=c_InPU*RoomWallAreas_NEWS(1,i);
c_Mid=c_MidPU*RoomWallAreas_NEWS(1,i);
c_Out=c_OutPU*RoomWallAreas_NEWS(1,i);

T_InWall=T_InWallNEWS(1,i);
T_MidWall=T_MidWallNEWS(1,i);
T_OutWall=T_OutWallNEWS(1,i);
    
aA=[-(k_InMid*RoomWallAreas_NEWS(1,i))/c_In (k_InMid*RoomWallAreas_NEWS(1,i))/c_In 0
 (k_InMid*RoomWallAreas_NEWS(1,i))/c_Mid -((k_InMid+k_OutMid)*RoomWallAreas_NEWS(1,i))/c_Mid (k_OutMid*RoomWallAreas_NEWS(1,i))/c_Mid
 0 (k_OutMid*RoomWallAreas_NEWS(1,i))/c_Out -(k_OutMid*RoomWallAreas_NEWS(1,i))/c_Out];

bA=[1/c_In 0 0
 0 1/c_Mid 0
 0 0 1/c_Out];
    
ab=[T_InWall
    T_MidWall
    T_OutWall];

bb=[(2.5*(T_Room-T_InWall)+5.6*(T_Room-T_InWall))*RoomWallAreas_NEWS(1,i)
0    
(2.8+3*v_Wind)*(T_Ambient-T_OutWall)+5.6*(T_Ambient-T_OutWall)*RoomWallAreas_NEWS(1,i)];

deltaT=aA*ab+bA*bb;

    deltaTint(1,i)=deltaT(1,1);
   deltaTmid(1,i)=deltaT(2,1);
    deltaTout(1,i)=deltaT(3,1);
    
    logRoomHeatLoss(1,i)=bb(1,1);
    
    else
        
        deltaTint(1,i)=0;
   deltaTmid(1,i)=0;
    deltaTout(1,i)=0;
        
    logRoomHeatLoss(1,i)=0;
    
    end
    
end

== matlab function Final_EWASP_VC/Subsystem_Room8/Bedroom3/Subsystem3/MATLAB Function ==
  data: uValWall input; deltaTint output; c_InPU input; c_MidPU input; c_OutPU input; T_InWall input; T_MidWall input; T_OutWall input; T_Room input; T_AmbientSeries input; windSpeedSeries input; deltaTmid output; deltaTout output; ceilArea input; roomNumber input; logRoomHeatLoss output; Time input; offsetDays input
function [deltaTint,deltaTmid,deltaTout,logRoomHeatLoss] = fcn(uValWall,c_InPU,c_MidPU,c_OutPU,T_InWall, T_MidWall,T_OutWall,T_Room,T_AmbientSeries,windSpeedSeries,ceilArea,roomNumber,Time,offsetDays)




  deltaTint=zeros(1,1);
   deltaTmid=zeros(1,1);
    deltaTout=zeros(1,1);
    logRoomHeatLoss=zeros(1,1);

    v_Wind=windSpeedSeries(ceil((offsetDays*1440)+Time/60+0.00001),1);
   T_Ambient=T_AmbientSeries(ceil((offsetDays*1440)+Time/60+0.00001),1);
    
k_InMid=uValWall*2;
k_OutMid=uValWall*2;




    
    if ceilArea>0

c_In=c_InPU*ceilArea;
c_Mid=c_MidPU*ceilArea;
c_Out=c_OutPU*ceilArea;

    
aA=[-(k_InMid*ceilArea)/c_In (k_InMid*ceilArea)/c_In 0
 (k_InMid*ceilArea)/c_Mid -((k_InMid+k_OutMid)*ceilArea)/c_Mid (k_OutMid*ceilArea)/c_Mid
 0 (k_OutMid*ceilArea)/c_Out -(k_OutMid*ceilArea)/c_Out];

bA=[1/c_In 0 0
 0 1/c_Mid 0
 0 0 1/c_Out];
    
ab=[T_InWall
    T_MidWall
    T_OutWall];

bb=[(2.5*(T_Room-T_InWall)+5.6*(T_Room-T_InWall))*ceilArea
0    
(2.8+3*v_Wind)*(T_Ambient-T_OutWall)+5.6*(T_Ambient-T_OutWall)*ceilArea];

deltaT=aA*ab+bA*bb;

    deltaTint=deltaT(1,1);
   deltaTmid=deltaT(2,1);
    deltaTout=deltaT(3,1);
    
    logRoomHeatLoss=bb(1,1);
    
    else
        
        deltaTint=0;
   deltaTmid=0;
    deltaTout=0;
        
    logRoomHeatLoss=0;
    
    end

== matlab function Final_EWASP_VC/Subsystem_Room8/Bedroom3/Subsystem3/MATLAB Function1 ==
  data: Time input; offsetDays input; SurfaceAlbedo input; Tot_Irradiance output; RoofArea input; c_OutRoof input; deltaTexternal output; RoofIrradiance input
function [Tot_Irradiance, deltaTexternal] = SolarSeriesToExtWallGains(Time,offsetDays,SurfaceAlbedo,RoofArea,c_OutRoof,RoofIrradiance)

PU_AreaIrr=RoofIrradiance(ceil((offsetDays*1440)+Time/60+0.00001),1)/2;%extracts correct Diff for the timestep, factor of 1/2 corrects for 90 degree walls (so only half Diff irradiance can be utilised)


Tot_Irradiance=(RoofArea*PU_AreaIrr)*(1-SurfaceAlbedo);
deltaTexternal=Tot_Irradiance./(c_OutRoof*RoofArea);

    
end

== matlab function Final_EWASP_VC/Subsystem_Room9/Bedroom4/Subsystem3/MATLAB Function ==
  data: uValWall input; deltaTint output; c_InPU input; c_MidPU input; c_OutPU input; T_InWall input; T_MidWall input; T_OutWall input; T_Room input; T_AmbientSeries input; windSpeedSeries input; deltaTmid output; deltaTout output; ceilArea input; roomNumber input; logRoomHeatLoss output; Time input; offsetDays input
function [deltaTint,deltaTmid,deltaTout,logRoomHeatLoss] = fcn(uValWall,c_InPU,c_MidPU,c_OutPU,T_InWall, T_MidWall,T_OutWall,T_Room,T_AmbientSeries,windSpeedSeries,ceilArea,roomNumber,Time,offsetDays)




  deltaTint=zeros(1,1);
   deltaTmid=zeros(1,1);
    deltaTout=zeros(1,1);
    logRoomHeatLoss=zeros(1,1);

    v_Wind=windSpeedSeries(ceil((offsetDays*1440)+Time/60+0.00001),1);
   T_Ambient=T_AmbientSeries(ceil((offsetDays*1440)+Time/60+0.00001),1);
    
k_InMid=uValWall*2;
k_OutMid=uValWall*2;




    
    if ceilArea>0

c_In=c_InPU*ceilArea;
c_Mid=c_MidPU*ceilArea;
c_Out=c_OutPU*ceilArea;

    
aA=[-(k_InMid*ceilArea)/c_In (k_InMid*ceilArea)/c_In 0
 (k_InMid*ceilArea)/c_Mid -((k_InMid+k_OutMid)*ceilArea)/c_Mid (k_OutMid*ceilArea)/c_Mid
 0 (k_OutMid*ceilArea)/c_Out -(k_OutMid*ceilArea)/c_Out];

bA=[1/c_In 0 0
 0 1/c_Mid 0
 0 0 1/c_Out];
    
ab=[T_InWall
    T_MidWall
    T_OutWall];

bb=[(2.5*(T_Room-T_InWall)+5.6*(T_Room-T_InWall))*ceilArea
0    
(2.8+3*v_Wind)*(T_Ambient-T_OutWall)+5.6*(T_Ambient-T_OutWall)*ceilArea];

deltaT=aA*ab+bA*bb;

    deltaTint=deltaT(1,1);
   deltaTmid=deltaT(2,1);
    deltaTout=deltaT(3,1);
    
    logRoomHeatLoss=bb(1,1);
    
    else
        
        deltaTint=0;
   deltaTmid=0;
    deltaTout=0;
        
    logRoomHeatLoss=0;
    
    end

== matlab function Final_EWASP_VC/Subsystem_Room9/Bedroom4/Subsystem3/MATLAB Function1 ==
  data: Time input; offsetDays input; SurfaceAlbedo input; Tot_Irradiance output; RoofArea input; c_OutRoof input; deltaTexternal output; RoofIrradiance input
function [Tot_Irradiance, deltaTexternal] = SolarSeriesToExtWallGains(Time,offsetDays,SurfaceAlbedo,RoofArea,c_OutRoof,RoofIrradiance)

PU_AreaIrr=RoofIrradiance(ceil((offsetDays*1440)+Time/60+0.00001),1)/2;%extracts correct Diff for the timestep, factor of 1/2 corrects for 90 degree walls (so only half Diff irradiance can be utilised)


Tot_Irradiance=(RoofArea*PU_AreaIrr)*(1-SurfaceAlbedo);
deltaTexternal=Tot_Irradiance./(c_OutRoof*RoofArea);

    
end

== matlab function Final_EWASP_VC/Subsystem_Room10/En suite/Subsystem3/MATLAB Function ==
  data: uValWall input; deltaTint output; c_InPU input; c_MidPU input; c_OutPU input; T_InWall input; T_MidWall input; T_OutWall input; T_Room input; T_AmbientSeries input; windSpeedSeries input; deltaTmid output; deltaTout output; ceilArea input; roomNumber input; logRoomHeatLoss output; Time input; offsetDays input
function [deltaTint,deltaTmid,deltaTout,logRoomHeatLoss] = fcn(uValWall,c_InPU,c_MidPU,c_OutPU,T_InWall, T_MidWall,T_OutWall,T_Room,T_AmbientSeries,windSpeedSeries,ceilArea,roomNumber,Time,offsetDays)




  deltaTint=zeros(1,1);
   deltaTmid=zeros(1,1);
    deltaTout=zeros(1,1);
    logRoomHeatLoss=zeros(1,1);

    v_Wind=windSpeedSeries(ceil((offsetDays*1440)+Time/60+0.00001),1);
   T_Ambient=T_AmbientSeries(ceil((offsetDays*1440)+Time/60+0.00001),1);
    
k_InMid=uValWall*2;
k_OutMid=uValWall*2;




    
    if ceilArea>0

c_In=c_InPU*ceilArea;
c_Mid=c_MidPU*ceilArea;
c_Out=c_OutPU*ceilArea;

    
aA=[-(k_InMid*ceilArea)/c_In (k_InMid*ceilArea)/c_In 0
 (k_InMid*ceilArea)/c_Mid -((k_InMid+k_OutMid)*ceilArea)/c_Mid (k_OutMid*ceilArea)/c_Mid
 0 (k_OutMid*ceilArea)/c_Out -(k_OutMid*ceilArea)/c_Out];

bA=[1/c_In 0 0
 0 1/c_Mid 0
 0 0 1/c_Out];
    
ab=[T_InWall
    T_MidWall
    T_OutWall];

bb=[(2.5*(T_Room-T_InWall)+5.6*(T_Room-T_InWall))*ceilArea
0    
(2.8+3*v_Wind)*(T_Ambient-T_OutWall)+5.6*(T_Ambient-T_OutWall)*ceilArea];

deltaT=aA*ab+bA*bb;

    deltaTint=deltaT(1,1);
   deltaTmid=deltaT(2,1);
    deltaTout=deltaT(3,1);
    
    logRoomHeatLoss=bb(1,1);
    
    else
        
        deltaTint=0;
   deltaTmid=0;
    deltaTout=0;
        
    logRoomHeatLoss=0;
    
    end

== matlab function Final_EWASP_VC/Subsystem_Room10/En suite/Subsystem3/MATLAB Function1 ==
  data: Time input; offsetDays input; SurfaceAlbedo input; Tot_Irradiance output; RoofArea input; c_OutRoof input; deltaTexternal output; RoofIrradiance input
function [Tot_Irradiance, deltaTexternal] = SolarSeriesToExtWallGains(Time,offsetDays,SurfaceAlbedo,RoofArea,c_OutRoof,RoofIrradiance)

PU_AreaIrr=RoofIrradiance(ceil((offsetDays*1440)+Time/60+0.00001),1)/2;%extracts correct Diff for the timestep, factor of 1/2 corrects for 90 degree walls (so only half Diff irradiance can be utilised)


Tot_Irradiance=(RoofArea*PU_AreaIrr)*(1-SurfaceAlbedo);
deltaTexternal=Tot_Irradiance./(c_OutRoof*RoofArea);

    
end

== matlab function Final_EWASP_VC/Subsystem_Room11/Bathroom/Subsystem3/MATLAB Function ==
  data: uValWall input; deltaTint output; c_InPU input; c_MidPU input; c_OutPU input; T_InWall input; T_MidWall input; T_OutWall input; T_Room input; T_AmbientSeries input; windSpeedSeries input; deltaTmid output; deltaTout output; ceilArea input; roomNumber input; logRoomHeatLoss output; Time input; offsetDays input
function [deltaTint,deltaTmid,deltaTout,logRoomHeatLoss] = fcn(uValWall,c_InPU,c_MidPU,c_OutPU,T_InWall, T_MidWall,T_OutWall,T_Room,T_AmbientSeries,windSpeedSeries,ceilArea,roomNumber,Time,offsetDays)




  deltaTint=zeros(1,1);
   deltaTmid=zeros(1,1);
    deltaTout=zeros(1,1);
    logRoomHeatLoss=zeros(1,1);

    v_Wind=windSpeedSeries(ceil((offsetDays*1440)+Time/60+0.00001),1);
   T_Ambient=T_AmbientSeries(ceil((offsetDays*1440)+Time/60+0.00001),1);
    
k_InMid=uValWall*2;
k_OutMid=uValWall*2;




    
    if ceilArea>0

c_In=c_InPU*ceilArea;
c_Mid=c_MidPU*ceilArea;
c_Out=c_OutPU*ceilArea;

    
aA=[-(k_InMid*ceilArea)/c_In (k_InMid*ceilArea)/c_In 0
 (k_InMid*ceilArea)/c_Mid -((k_InMid+k_OutMid)*ceilArea)/c_Mid (k_OutMid*ceilArea)/c_Mid
 0 (k_OutMid*ceilArea)/c_Out -(k_OutMid*ceilArea)/c_Out];

bA=[1/c_In 0 0
 0 1/c_Mid 0
 0 0 1/c_Out];
    
ab=[T_InWall
    T_MidWall
    T_OutWall];

bb=[(2.5*(T_Room-T_InWall)+5.6*(T_Room-T_InWall))*ceilArea
0    
(2.8+3*v_Wind)*(T_Ambient-T_OutWall)+5.6*(T_Ambient-T_OutWall)*ceilArea];

deltaT=aA*ab+bA*bb;

    deltaTint=deltaT(1,1);
   deltaTmid=deltaT(2,1);
    deltaTout=deltaT(3,1);
    
    logRoomHeatLoss=bb(1,1);
    
    else
        
        deltaTint=0;
   deltaTmid=0;
    deltaTout=0;
        
    logRoomHeatLoss=0;
    
    end
